simulink model "waterTankBurner"  (R2014b)
settings: Solver=ode1  StartTime=0.0  StopTime=100  FixedStep=0.0001  MaxStep=0.0001  RelTol=1e-3
(part 1 of 4)
settings Model: Creator=sand080  LastModifiedBy=nall426
settings DataIOCC: LimitDataPoints=off
settings RTWCC: CustomInitializer=gettimeofday(&t0, 0);
settings RTWCC: CustomSourceCode=|
  | int gettimeofday(struct timeval * tp, struct timezone * tzp)
  | {
  |     // Note: some broken versions only have 8 trailing zero's, the correct epoch has 9 trailing zero's
  |     static const uint64_t EPOCH = ((uint64_t) 116444736000000000ULL);
  | 
  |     SYSTEMTIME  system_time;
  |     FILETIME    file_time;
  |     uint64_t    time;
  | 
  | 	GetSystemTime( &system_time );
  |     SystemTimeToFileTime( &system_time, &file_time );
  |     time =  ((uint64_t)file_time.dwLowDateTime )      ;
  |     time += ((uint64_t)file_time.dwHighDateTime) << 32;
  | 
  |     tp->tv_sec  = (long) ((time - EPOCH) / 10000000L);
  |     tp->tv_usec = (long) (system_time.wMilliseconds * 1000);
  |     return 0;
  | }
  | 
  | struct timeval t0, t1;
settings RTWCC: CustomHeaderCode=|
  | #include <stdint.h> // portable: uint64_t   MSVC: __int64
  | #include <Windows.h>
settings RTWCC: CustomTerminator=|
  | gettimeofday(&t1, 0);
  | 
  | long elapsed = (t1.tv_sec-t0.tv_sec)*1000000 + t1.tv_usec-t0.tv_usec;
  | printf("Time taken: %ld microseconds (%.3f seconds)\n", elapsed, (elapsed / 1000000.0));

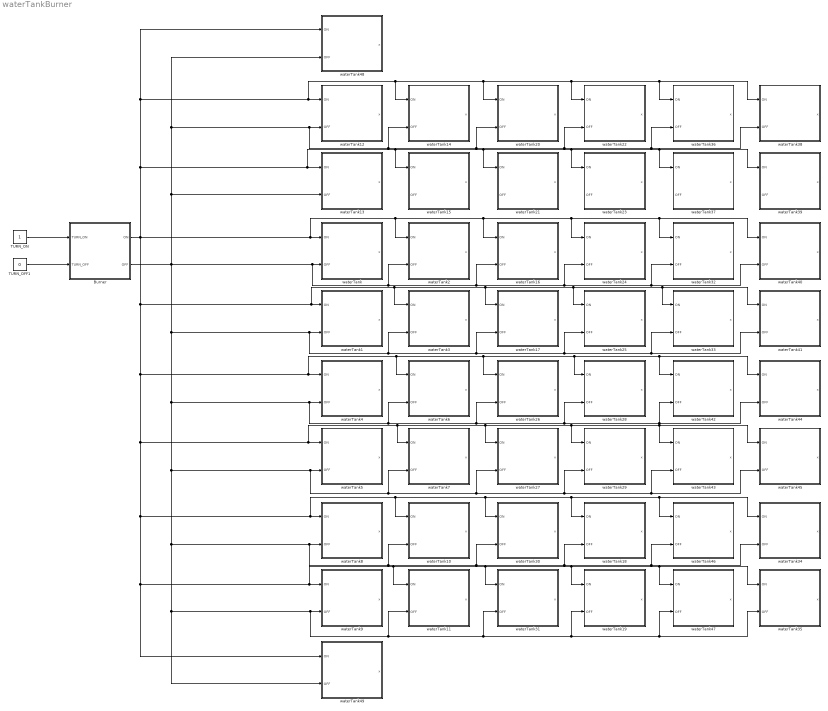
== system waterTankBurner ==
  Burner : Subsystem
  TURN_OFF1 : Constant  Value=0
  TURN_ON : Constant
  waterTank : Subsystem
  waterTank1 : Subsystem
  waterTank10 : Subsystem
  waterTank11 : Subsystem
  waterTank12 : Subsystem
  waterTank13 : Subsystem
  waterTank14 : Subsystem
  waterTank15 : Subsystem
  waterTank16 : Subsystem
  waterTank17 : Subsystem
  waterTank18 : Subsystem
  waterTank19 : Subsystem
  waterTank2 : Subsystem
  waterTank20 : Subsystem
  waterTank21 : Subsystem
  waterTank22 : Subsystem
  waterTank23 : Subsystem
  waterTank24 : Subsystem
  waterTank25 : Subsystem
  waterTank26 : Subsystem
  waterTank27 : Subsystem
  waterTank28 : Subsystem
  waterTank29 : Subsystem
  waterTank3 : Subsystem
  waterTank30 : Subsystem
  waterTank31 : Subsystem
  waterTank32 : Subsystem
  waterTank33 : Subsystem
  waterTank34 : Subsystem
  waterTank35 : Subsystem
  waterTank36 : Subsystem
  waterTank37 : Subsystem
  waterTank38 : Subsystem
  waterTank39 : Subsystem
  waterTank4 : Subsystem
  waterTank40 : Subsystem
  waterTank41 : Subsystem
  waterTank42 : Subsystem
  waterTank43 : Subsystem
  waterTank44 : Subsystem
  waterTank45 : Subsystem
  waterTank46 : Subsystem
  waterTank47 : Subsystem
  waterTank48 : Subsystem
  waterTank49 : Subsystem
  waterTank5 : Subsystem
  waterTank6 : Subsystem
  waterTank7 : Subsystem
  waterTank8 : Subsystem
  waterTank9 : Subsystem
  wires:
  TURN_ON/1 -> Burner/1(TURN_ON)
  TURN_OFF1/1 -> Burner/2(TURN_OFF)
  Burner/1(ON) -> waterTank38/1(ON), waterTank36/1(ON), waterTank22/1(ON), waterTank20/1(ON), waterTank14/1(ON), waterTank12/1(ON), waterTank48/1(ON), waterTank39/1(ON), waterTank37/1(ON), waterTank23/1(ON), waterTank21/1(ON), waterTank15/1(ON), waterTank13/1(ON), waterTank49/1(ON), waterTank11/1(ON), waterTank31/1(ON), waterTank19/1(ON), waterTank47/1(ON), waterTank35/1(ON), waterTank9/1(ON), waterTank10/1(ON), waterTank30/1(ON), waterTank18/1(ON), waterTank46/1(ON), waterTank34/1(ON), waterTank8/1(ON), waterTank7/1(ON), waterTank27/1(ON), waterTank29/1(ON), waterTank43/1(ON), waterTank45/1(ON), waterTank5/1(ON), waterTank6/1(ON), waterTank26/1(ON), waterTank28/1(ON), waterTank42/1(ON), waterTank44/1(ON), waterTank4/1(ON), waterTank3/1(ON), waterTank25/1(ON), waterTank33/1(ON), waterTank41/1(ON), waterTank17/1(ON), waterTank1/1(ON), waterTank40/1(ON), waterTank32/1(ON), waterTank24/1(ON), waterTank16/1(ON), waterTank2/1(ON), waterTank/1(ON)
  Burner/2(OFF) -> waterTank48/2(OFF), waterTank36/2(OFF), waterTank38/2(OFF), waterTank22/2(OFF), waterTank20/2(OFF), waterTank14/2(OFF), waterTank12/2(OFF), waterTank13/2(OFF), waterTank49/2(OFF), waterTank19/2(OFF), waterTank47/2(OFF), waterTank35/2(OFF), waterTank31/2(OFF), waterTank11/2(OFF), waterTank9/2(OFF), waterTank46/2(OFF), waterTank34/2(OFF), waterTank18/2(OFF), waterTank30/2(OFF), waterTank10/2(OFF), waterTank8/2(OFF), waterTank43/2(OFF), waterTank45/2(OFF), waterTank29/2(OFF), waterTank27/2(OFF), waterTank7/2(OFF), waterTank5/2(OFF), waterTank42/2(OFF), waterTank44/2(OFF), waterTank28/2(OFF), waterTank26/2(OFF), waterTank6/2(OFF), waterTank4/2(OFF), waterTank33/2(OFF), waterTank41/2(OFF), waterTank25/2(OFF), waterTank17/2(OFF), waterTank3/2(OFF), waterTank1/2(OFF), waterTank16/2(OFF), waterTank40/2(OFF), waterTank32/2(OFF), waterTank24/2(OFF), waterTank2/2(OFF), waterTank/2(OFF)

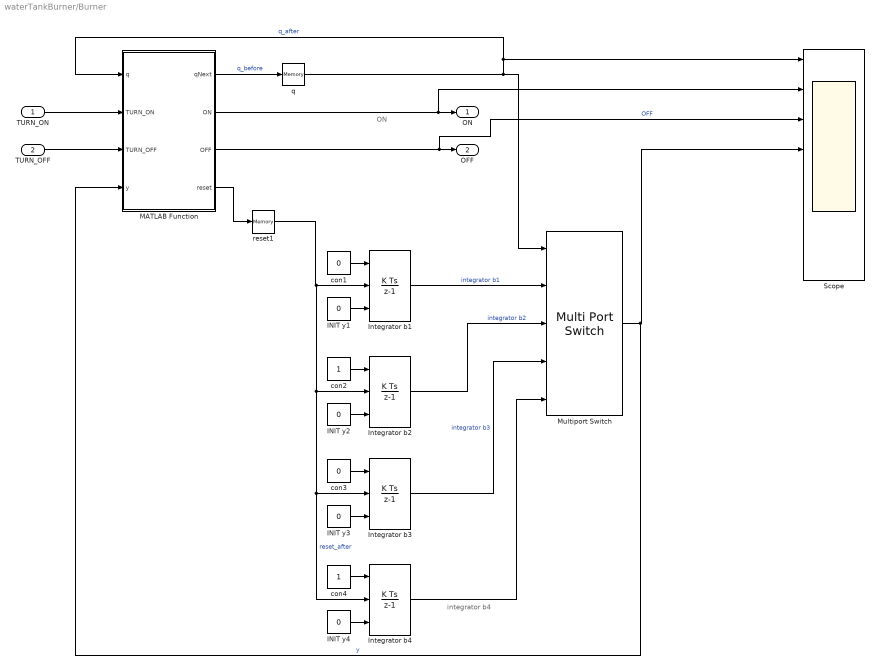
== system waterTankBurner/Burner ==
  note: integrator b4
  note: ON
  TURN_ON : Inport
  TURN_OFF : Inport  Port=2
  INIT y{1..4} (4 alike) : Constant  Value=0
  Integrator b{1..4} (4 alike) : DiscreteIntegrator  ExternalReset=either  InitialConditionSource=external  InitialCondition=510  InitialConditionSetting=State (most efficient)  SampleTime=-1
  MATLAB Function : MATLAB Function  Priority=1  TreatAsAtomicUnit=on
  Multiport Switch : MultiPortSwitch  Inputs=4
  Scope : Scope  NumInputPorts=8
      settings: TickLabels=on  ShowLegends=on  YMin=0~0~0~0~0~0~0~0  YMax=1~1~1~1~1~1~1~1
  con1 : Constant  Value=0
  con2 : Constant
  con3 : Constant  Value=0
  con4 : Constant
  q : Memory  X0=1  LinearizeMemory=on
  reset1 : Memory  LinearizeMemory=on
  ON : Outport
  OFF : Outport  Port=2
  wires:
  MATLAB Function/3(OFF) -> Scope/3, OFF/1  "OFF"
  INIT y1/1 -> Integrator b1/3
  INIT y2/1 -> Integrator b2/3
  con1/1 -> Integrator b1/1
  MATLAB Function/1(qNext) -> q/1  "q_before"
  q/1 -> Multiport Switch/1, MATLAB Function/1(q), Scope/1  "q_after"
  MATLAB Function/4(reset) -> reset1/1
  con2/1 -> Integrator b2/1
  MATLAB Function/2(ON) -> Scope/2, ON/1
  TURN_OFF/1 -> MATLAB Function/3(TURN_OFF)
  TURN_ON/1 -> MATLAB Function/2(TURN_ON)
  INIT y3/1 -> Integrator b3/3
  INIT y4/1 -> Integrator b4/3
  con3/1 -> Integrator b3/1
  con4/1 -> Integrator b4/1
  reset1/1 -> Integrator b4/2, Integrator b3/2, Integrator b2/2, Integrator b1/2  "reset_after"
  Integrator b1/1 -> Multiport Switch/2  "integrator b1"
  Integrator b2/1 -> Multiport Switch/3  "integrator b2"
  Integrator b3/1 -> Multiport Switch/4  "integrator b3"
  Integrator b4/1 -> Multiport Switch/5
  Multiport Switch/1 -> MATLAB Function/4(y), Scope/4  "y"

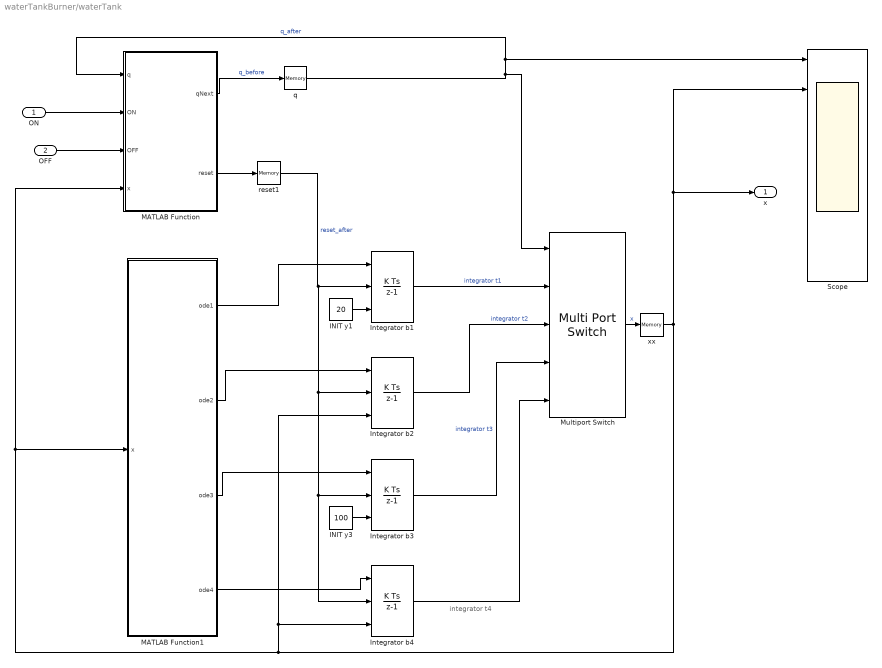
== system waterTankBurner/waterTank ==
  note: integrator t4
  ON : Inport
  OFF : Inport  Port=2
  INIT y1 : Constant  Value=20
  INIT y3 : Constant  Value=100
  Integrator b{1..4} (4 alike) : DiscreteIntegrator  ExternalReset=either  InitialConditionSource=external  InitialCondition=510  InitialConditionSetting=State (most efficient)  SampleTime=-1
  MATLAB Function : MATLAB Function  Priority=1  TreatAsAtomicUnit=on
  MATLAB Function1 : MATLAB Function  TreatAsAtomicUnit=on
  Multiport Switch : MultiPortSwitch  Inputs=4
  Scope : Scope  NumInputPorts=8
      settings: TickLabels=on  ShowLegends=on  YMin=0~0~0~0~0~0~0~0  YMax=1~1~1~1~1~1~1~1
  q : Memory  X0=1  LinearizeMemory=on
  reset1 : Memory  LinearizeMemory=on
  xx : Memory  LinearizeMemory=on
  x : Outport
  wires:
  INIT y1/1 -> Integrator b1/3
  MATLAB Function1/1(ode1) -> Integrator b1/1
  MATLAB Function/1(qNext) -> q/1  "q_before"
  q/1 -> Multiport Switch/1, MATLAB Function/1(q), Scope/1  "q_after"
  MATLAB Function/2(reset) -> reset1/1
  MATLAB Function1/2(ode2) -> Integrator b2/1
  INIT y3/1 -> Integrator b3/3
  MATLAB Function1/3(ode3) -> Integrator b3/1
  MATLAB Function1/4(ode4) -> Integrator b4/1
  reset1/1 -> Integrator b4/2, Integrator b3/2, Integrator b2/2, Integrator b1/2  "reset_after"
  Integrator b1/1 -> Multiport Switch/2  "integrator t1"
  Integrator b2/1 -> Multiport Switch/3  "integrator t2"
  Integrator b3/1 -> Multiport Switch/4  "integrator t3"
  Integrator b4/1 -> Multiport Switch/5
  OFF/1 -> MATLAB Function/3(OFF)
  ON/1 -> MATLAB Function/2(ON)
  xx/1 -> x/1, Scope/2, Integrator b2/3, Integrator b4/3, MATLAB Function1/1(x), MATLAB Function/4(x)
  Multiport Switch/1 -> xx/1  "x"

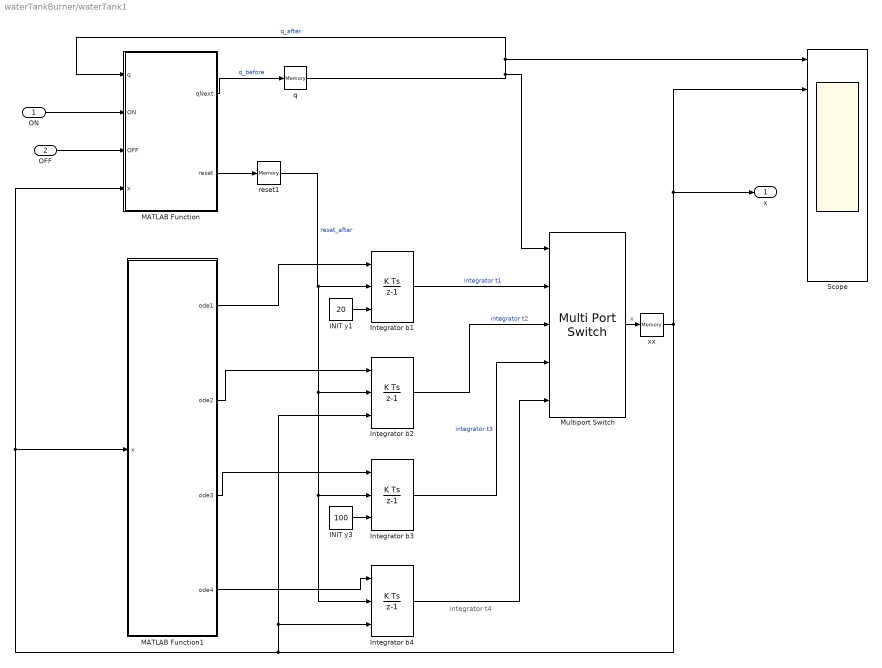
== system waterTankBurner/waterTank1 ==
  note: integrator t4
  ON : Inport
  OFF : Inport  Port=2
  INIT y1 : Constant  Value=20
  INIT y3 : Constant  Value=100
  Integrator b{1..4} (4 alike) : DiscreteIntegrator  ExternalReset=either  InitialConditionSource=external  InitialCondition=510  InitialConditionSetting=State (most efficient)  SampleTime=-1
  MATLAB Function : MATLAB Function  Priority=1  TreatAsAtomicUnit=on
  MATLAB Function1 : MATLAB Function  TreatAsAtomicUnit=on
  Multiport Switch : MultiPortSwitch  Inputs=4
  Scope : Scope  NumInputPorts=8
      settings: TickLabels=on  ShowLegends=on  YMin=0~0~0~0~0~0~0~0  YMax=1~1~1~1~1~1~1~1
  q : Memory  X0=1  LinearizeMemory=on
  reset1 : Memory  LinearizeMemory=on
  xx : Memory  LinearizeMemory=on
  x : Outport
  wires:
  INIT y1/1 -> Integrator b1/3
  MATLAB Function1/1(ode1) -> Integrator b1/1
  MATLAB Function/1(qNext) -> q/1  "q_before"
  q/1 -> Multiport Switch/1, MATLAB Function/1(q), Scope/1  "q_after"
  MATLAB Function/2(reset) -> reset1/1
  MATLAB Function1/2(ode2) -> Integrator b2/1
  INIT y3/1 -> Integrator b3/3
  MATLAB Function1/3(ode3) -> Integrator b3/1
  MATLAB Function1/4(ode4) -> Integrator b4/1
  reset1/1 -> Integrator b4/2, Integrator b3/2, Integrator b2/2, Integrator b1/2  "reset_after"
  Integrator b1/1 -> Multiport Switch/2  "integrator t1"
  Integrator b2/1 -> Multiport Switch/3  "integrator t2"
  Integrator b3/1 -> Multiport Switch/4  "integrator t3"
  Integrator b4/1 -> Multiport Switch/5
  OFF/1 -> MATLAB Function/3(OFF)
  ON/1 -> MATLAB Function/2(ON)
  xx/1 -> x/1, Scope/2, Integrator b2/3, Integrator b4/3, MATLAB Function1/1(x), MATLAB Function/4(x)
  Multiport Switch/1 -> xx/1  "x"

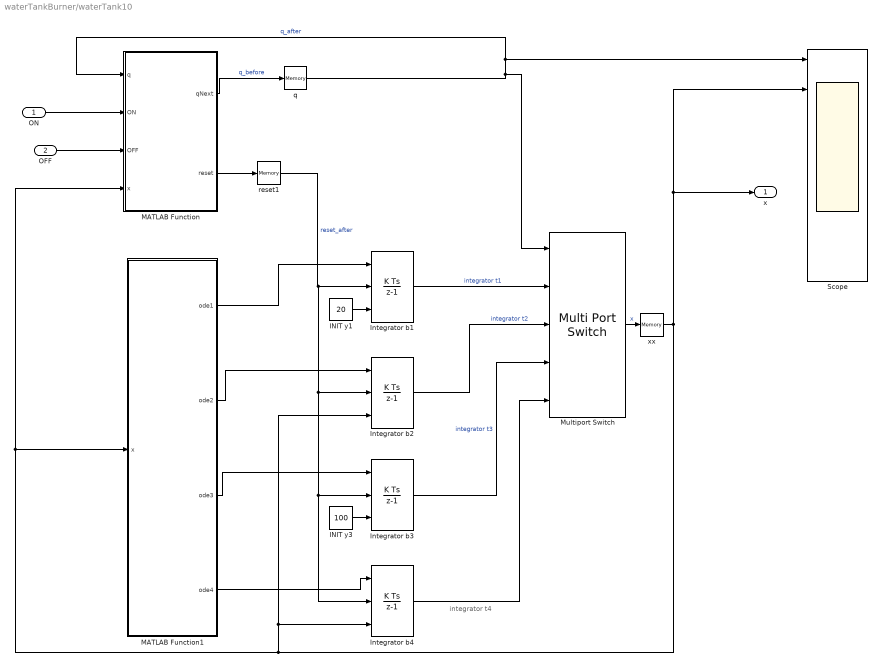
== system waterTankBurner/waterTank10 ==
  note: integrator t4
  ON : Inport
  OFF : Inport  Port=2
  INIT y1 : Constant  Value=20
  INIT y3 : Constant  Value=100
  Integrator b{1..4} (4 alike) : DiscreteIntegrator  ExternalReset=either  InitialConditionSource=external  InitialCondition=510  InitialConditionSetting=State (most efficient)  SampleTime=-1
  MATLAB Function : MATLAB Function  Priority=1  TreatAsAtomicUnit=on
  MATLAB Function1 : MATLAB Function  TreatAsAtomicUnit=on
  Multiport Switch : MultiPortSwitch  Inputs=4
  Scope : Scope  NumInputPorts=8
      settings: TickLabels=on  ShowLegends=on  YMin=0~0~0~0~0~0~0~0  YMax=1~1~1~1~1~1~1~1
  q : Memory  X0=1  LinearizeMemory=on
  reset1 : Memory  LinearizeMemory=on
  xx : Memory  LinearizeMemory=on
  x : Outport
  wires:
  INIT y1/1 -> Integrator b1/3
  MATLAB Function1/1(ode1) -> Integrator b1/1
  MATLAB Function/1(qNext) -> q/1  "q_before"
  q/1 -> Multiport Switch/1, MATLAB Function/1(q), Scope/1  "q_after"
  MATLAB Function/2(reset) -> reset1/1
  MATLAB Function1/2(ode2) -> Integrator b2/1
  INIT y3/1 -> Integrator b3/3
  MATLAB Function1/3(ode3) -> Integrator b3/1
  MATLAB Function1/4(ode4) -> Integrator b4/1
  reset1/1 -> Integrator b4/2, Integrator b3/2, Integrator b2/2, Integrator b1/2  "reset_after"
  Integrator b1/1 -> Multiport Switch/2  "integrator t1"
  Integrator b2/1 -> Multiport Switch/3  "integrator t2"
  Integrator b3/1 -> Multiport Switch/4  "integrator t3"
  Integrator b4/1 -> Multiport Switch/5
  OFF/1 -> MATLAB Function/3(OFF)
  ON/1 -> MATLAB Function/2(ON)
  xx/1 -> x/1, Scope/2, Integrator b2/3, Integrator b4/3, MATLAB Function1/1(x), MATLAB Function/4(x)
  Multiport Switch/1 -> xx/1  "x"

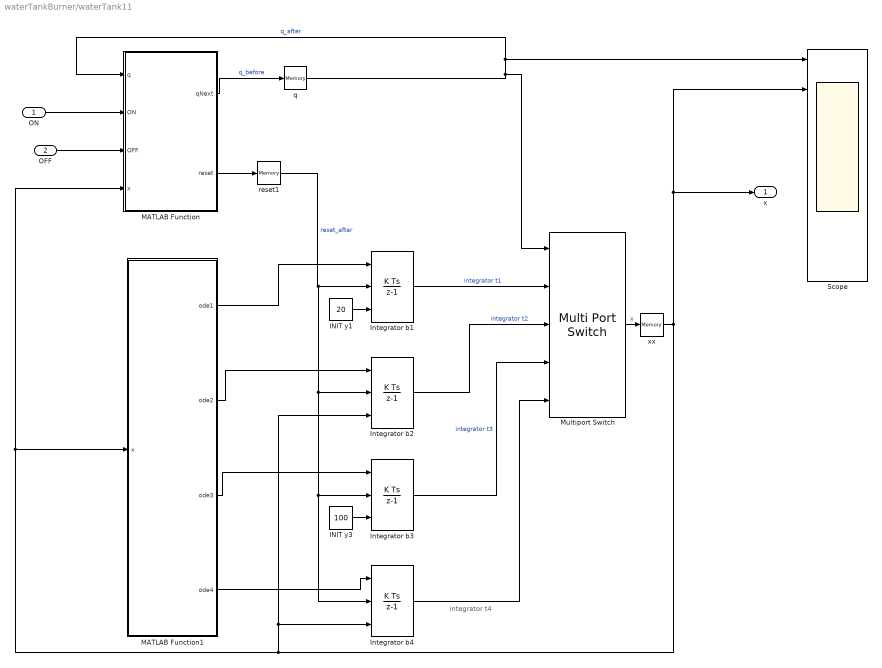
== system waterTankBurner/waterTank11 ==
  note: integrator t4
  ON : Inport
  OFF : Inport  Port=2
  INIT y1 : Constant  Value=20
  INIT y3 : Constant  Value=100
  Integrator b{1..4} (4 alike) : DiscreteIntegrator  ExternalReset=either  InitialConditionSource=external  InitialCondition=510  InitialConditionSetting=State (most efficient)  SampleTime=-1
  MATLAB Function : MATLAB Function  Priority=1  TreatAsAtomicUnit=on
  MATLAB Function1 : MATLAB Function  TreatAsAtomicUnit=on
  Multiport Switch : MultiPortSwitch  Inputs=4
  Scope : Scope  NumInputPorts=8
      settings: TickLabels=on  ShowLegends=on  YMin=0~0~0~0~0~0~0~0  YMax=1~1~1~1~1~1~1~1
  q : Memory  X0=1  LinearizeMemory=on
  reset1 : Memory  LinearizeMemory=on
  xx : Memory  LinearizeMemory=on
  x : Outport
  wires:
  INIT y1/1 -> Integrator b1/3
  MATLAB Function1/1(ode1) -> Integrator b1/1
  MATLAB Function/1(qNext) -> q/1  "q_before"
  q/1 -> Multiport Switch/1, MATLAB Function/1(q), Scope/1  "q_after"
  MATLAB Function/2(reset) -> reset1/1
  MATLAB Function1/2(ode2) -> Integrator b2/1
  INIT y3/1 -> Integrator b3/3
  MATLAB Function1/3(ode3) -> Integrator b3/1
  MATLAB Function1/4(ode4) -> Integrator b4/1
  reset1/1 -> Integrator b4/2, Integrator b3/2, Integrator b2/2, Integrator b1/2  "reset_after"
  Integrator b1/1 -> Multiport Switch/2  "integrator t1"
  Integrator b2/1 -> Multiport Switch/3  "integrator t2"
  Integrator b3/1 -> Multiport Switch/4  "integrator t3"
  Integrator b4/1 -> Multiport Switch/5
  OFF/1 -> MATLAB Function/3(OFF)
  ON/1 -> MATLAB Function/2(ON)
  xx/1 -> x/1, Scope/2, Integrator b2/3, Integrator b4/3, MATLAB Function1/1(x), MATLAB Function/4(x)
  Multiport Switch/1 -> xx/1  "x"

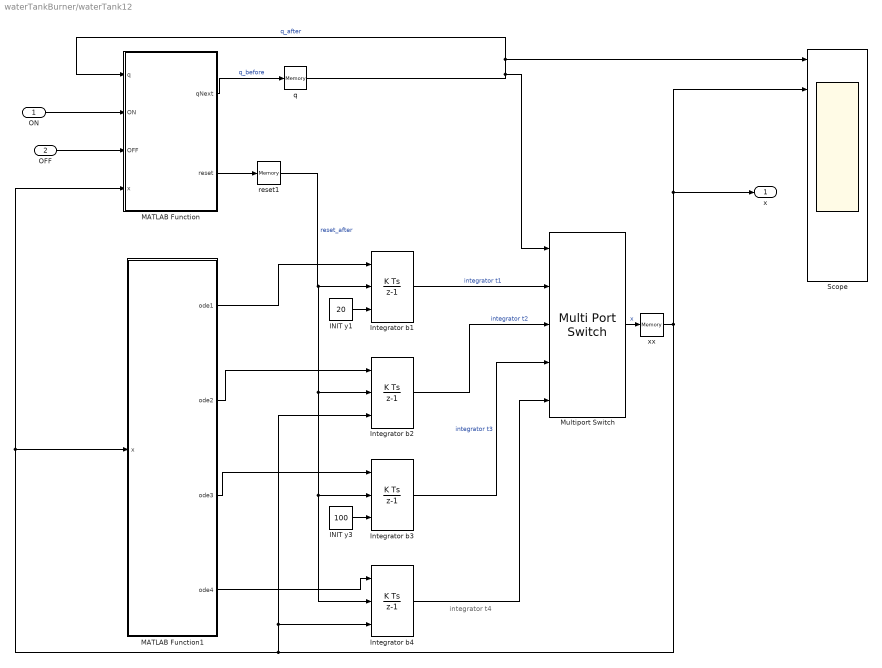
== system waterTankBurner/waterTank12 ==
  note: integrator t4
  ON : Inport
  OFF : Inport  Port=2
  INIT y1 : Constant  Value=20
  INIT y3 : Constant  Value=100
  Integrator b{1..4} (4 alike) : DiscreteIntegrator  ExternalReset=either  InitialConditionSource=external  InitialCondition=510  InitialConditionSetting=State (most efficient)  SampleTime=-1
  MATLAB Function : MATLAB Function  Priority=1  TreatAsAtomicUnit=on
  MATLAB Function1 : MATLAB Function  TreatAsAtomicUnit=on
  Multiport Switch : MultiPortSwitch  Inputs=4
  Scope : Scope  NumInputPorts=8
      settings: TickLabels=on  ShowLegends=on  YMin=0~0~0~0~0~0~0~0  YMax=1~1~1~1~1~1~1~1
  q : Memory  X0=1  LinearizeMemory=on
  reset1 : Memory  LinearizeMemory=on
  xx : Memory  LinearizeMemory=on
  x : Outport
  wires:
  INIT y1/1 -> Integrator b1/3
  MATLAB Function1/1(ode1) -> Integrator b1/1
  MATLAB Function/1(qNext) -> q/1  "q_before"
  q/1 -> Multiport Switch/1, MATLAB Function/1(q), Scope/1  "q_after"
  MATLAB Function/2(reset) -> reset1/1
  MATLAB Function1/2(ode2) -> Integrator b2/1
  INIT y3/1 -> Integrator b3/3
  MATLAB Function1/3(ode3) -> Integrator b3/1
  MATLAB Function1/4(ode4) -> Integrator b4/1
  reset1/1 -> Integrator b4/2, Integrator b3/2, Integrator b2/2, Integrator b1/2  "reset_after"
  Integrator b1/1 -> Multiport Switch/2  "integrator t1"
  Integrator b2/1 -> Multiport Switch/3  "integrator t2"
  Integrator b3/1 -> Multiport Switch/4  "integrator t3"
  Integrator b4/1 -> Multiport Switch/5
  OFF/1 -> MATLAB Function/3(OFF)
  ON/1 -> MATLAB Function/2(ON)
  xx/1 -> x/1, Scope/2, Integrator b2/3, Integrator b4/3, MATLAB Function1/1(x), MATLAB Function/4(x)
  Multiport Switch/1 -> xx/1  "x"

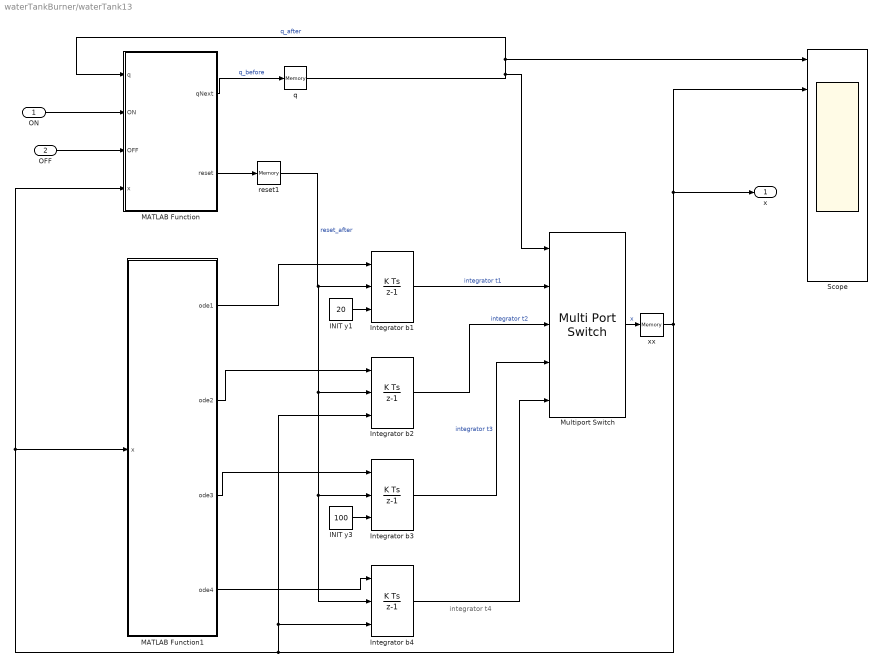
== system waterTankBurner/waterTank13 ==
  note: integrator t4
  ON : Inport
  OFF : Inport  Port=2
  INIT y1 : Constant  Value=20
  INIT y3 : Constant  Value=100
  Integrator b{1..4} (4 alike) : DiscreteIntegrator  ExternalReset=either  InitialConditionSource=external  InitialCondition=510  InitialConditionSetting=State (most efficient)  SampleTime=-1
  MATLAB Function : MATLAB Function  Priority=1  TreatAsAtomicUnit=on
  MATLAB Function1 : MATLAB Function  TreatAsAtomicUnit=on
  Multiport Switch : MultiPortSwitch  Inputs=4
  Scope : Scope  NumInputPorts=8
      settings: TickLabels=on  ShowLegends=on  YMin=0~0~0~0~0~0~0~0  YMax=1~1~1~1~1~1~1~1
  q : Memory  X0=1  LinearizeMemory=on
  reset1 : Memory  LinearizeMemory=on
  xx : Memory  LinearizeMemory=on
  x : Outport
  wires:
  INIT y1/1 -> Integrator b1/3
  MATLAB Function1/1(ode1) -> Integrator b1/1
  MATLAB Function/1(qNext) -> q/1  "q_before"
  q/1 -> Multiport Switch/1, MATLAB Function/1(q), Scope/1  "q_after"
  MATLAB Function/2(reset) -> reset1/1
  MATLAB Function1/2(ode2) -> Integrator b2/1
  INIT y3/1 -> Integrator b3/3
  MATLAB Function1/3(ode3) -> Integrator b3/1
  MATLAB Function1/4(ode4) -> Integrator b4/1
  reset1/1 -> Integrator b4/2, Integrator b3/2, Integrator b2/2, Integrator b1/2  "reset_after"
  Integrator b1/1 -> Multiport Switch/2  "integrator t1"
  Integrator b2/1 -> Multiport Switch/3  "integrator t2"
  Integrator b3/1 -> Multiport Switch/4  "integrator t3"
  Integrator b4/1 -> Multiport Switch/5
  OFF/1 -> MATLAB Function/3(OFF)
  ON/1 -> MATLAB Function/2(ON)
  xx/1 -> x/1, Scope/2, Integrator b2/3, Integrator b4/3, MATLAB Function1/1(x), MATLAB Function/4(x)
  Multiport Switch/1 -> xx/1  "x"

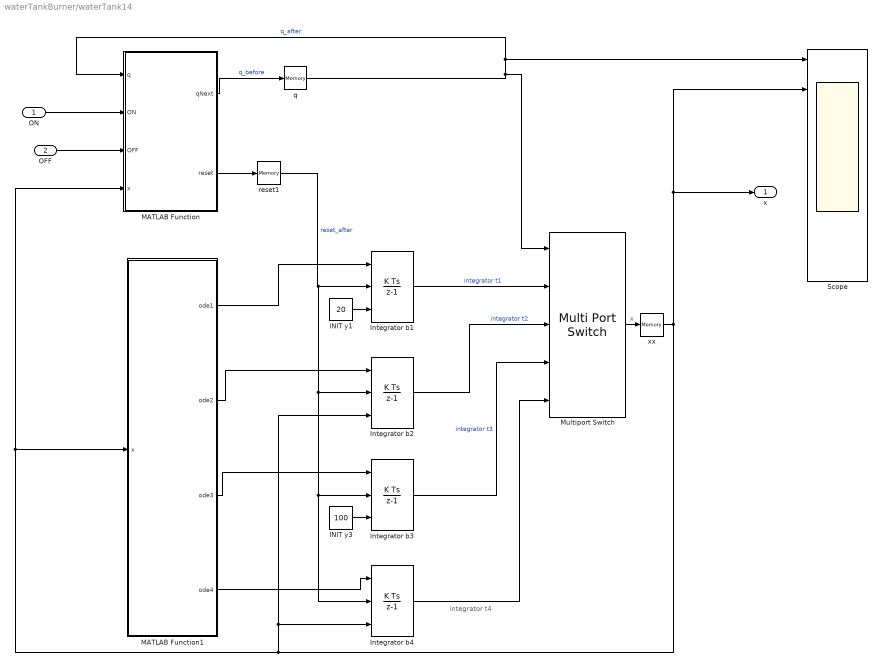
== system waterTankBurner/waterTank14 ==
  note: integrator t4
  ON : Inport
  OFF : Inport  Port=2
  INIT y1 : Constant  Value=20
  INIT y3 : Constant  Value=100
  Integrator b{1..4} (4 alike) : DiscreteIntegrator  ExternalReset=either  InitialConditionSource=external  InitialCondition=510  InitialConditionSetting=State (most efficient)  SampleTime=-1
  MATLAB Function : MATLAB Function  Priority=1  TreatAsAtomicUnit=on
  MATLAB Function1 : MATLAB Function  TreatAsAtomicUnit=on
  Multiport Switch : MultiPortSwitch  Inputs=4
  Scope : Scope  NumInputPorts=8
      settings: TickLabels=on  ShowLegends=on  YMin=0~0~0~0~0~0~0~0  YMax=1~1~1~1~1~1~1~1
  q : Memory  X0=1  LinearizeMemory=on
  reset1 : Memory  LinearizeMemory=on
  xx : Memory  LinearizeMemory=on
  x : Outport
  wires:
  INIT y1/1 -> Integrator b1/3
  MATLAB Function1/1(ode1) -> Integrator b1/1
  MATLAB Function/1(qNext) -> q/1  "q_before"
  q/1 -> Multiport Switch/1, MATLAB Function/1(q), Scope/1  "q_after"
  MATLAB Function/2(reset) -> reset1/1
  MATLAB Function1/2(ode2) -> Integrator b2/1
  INIT y3/1 -> Integrator b3/3
  MATLAB Function1/3(ode3) -> Integrator b3/1
  MATLAB Function1/4(ode4) -> Integrator b4/1
  reset1/1 -> Integrator b4/2, Integrator b3/2, Integrator b2/2, Integrator b1/2  "reset_after"
  Integrator b1/1 -> Multiport Switch/2  "integrator t1"
  Integrator b2/1 -> Multiport Switch/3  "integrator t2"
  Integrator b3/1 -> Multiport Switch/4  "integrator t3"
  Integrator b4/1 -> Multiport Switch/5
  OFF/1 -> MATLAB Function/3(OFF)
  ON/1 -> MATLAB Function/2(ON)
  xx/1 -> x/1, Scope/2, Integrator b2/3, Integrator b4/3, MATLAB Function1/1(x), MATLAB Function/4(x)
  Multiport Switch/1 -> xx/1  "x"

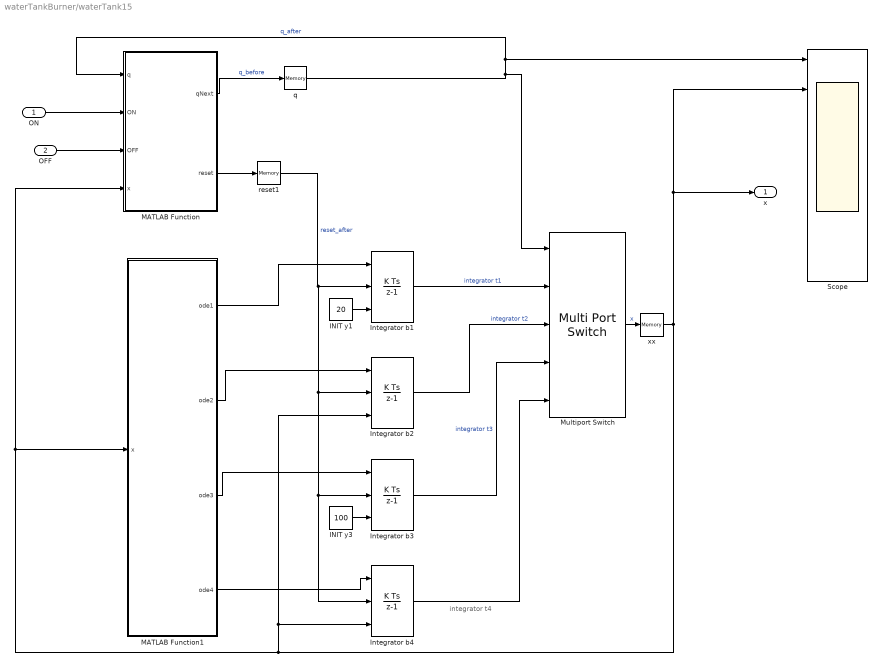
== system waterTankBurner/waterTank15 ==
  note: integrator t4
  ON : Inport
  OFF : Inport  Port=2
  INIT y1 : Constant  Value=20
  INIT y3 : Constant  Value=100
  Integrator b{1..4} (4 alike) : DiscreteIntegrator  ExternalReset=either  InitialConditionSource=external  InitialCondition=510  InitialConditionSetting=State (most efficient)  SampleTime=-1
  MATLAB Function : MATLAB Function  Priority=1  TreatAsAtomicUnit=on
  MATLAB Function1 : MATLAB Function  TreatAsAtomicUnit=on
  Multiport Switch : MultiPortSwitch  Inputs=4
  Scope : Scope  NumInputPorts=8
      settings: TickLabels=on  ShowLegends=on  YMin=0~0~0~0~0~0~0~0  YMax=1~1~1~1~1~1~1~1
  q : Memory  X0=1  LinearizeMemory=on
  reset1 : Memory  LinearizeMemory=on
  xx : Memory  LinearizeMemory=on
  x : Outport
  wires:
  INIT y1/1 -> Integrator b1/3
  MATLAB Function1/1(ode1) -> Integrator b1/1
  MATLAB Function/1(qNext) -> q/1  "q_before"
  q/1 -> Multiport Switch/1, MATLAB Function/1(q), Scope/1  "q_after"
  MATLAB Function/2(reset) -> reset1/1
  MATLAB Function1/2(ode2) -> Integrator b2/1
  INIT y3/1 -> Integrator b3/3
  MATLAB Function1/3(ode3) -> Integrator b3/1
  MATLAB Function1/4(ode4) -> Integrator b4/1
  reset1/1 -> Integrator b4/2, Integrator b3/2, Integrator b2/2, Integrator b1/2  "reset_after"
  Integrator b1/1 -> Multiport Switch/2  "integrator t1"
  Integrator b2/1 -> Multiport Switch/3  "integrator t2"
  Integrator b3/1 -> Multiport Switch/4  "integrator t3"
  Integrator b4/1 -> Multiport Switch/5
  OFF/1 -> MATLAB Function/3(OFF)
  ON/1 -> MATLAB Function/2(ON)
  xx/1 -> x/1, Scope/2, Integrator b2/3, Integrator b4/3, MATLAB Function1/1(x), MATLAB Function/4(x)
  Multiport Switch/1 -> xx/1  "x"

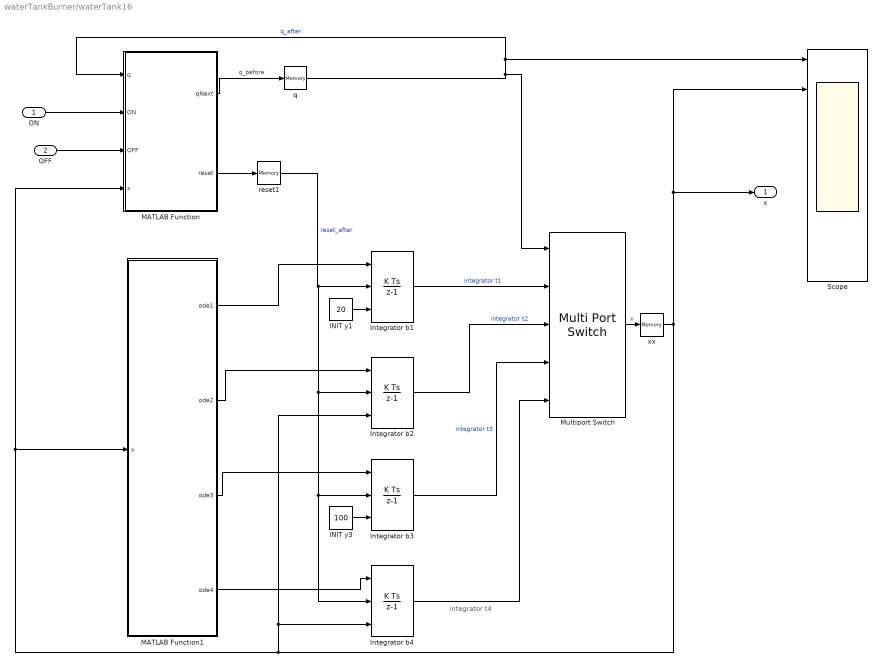
== system waterTankBurner/waterTank16 ==
  note: integrator t4
  ON : Inport
  OFF : Inport  Port=2
  INIT y1 : Constant  Value=20
  INIT y3 : Constant  Value=100
  Integrator b{1..4} (4 alike) : DiscreteIntegrator  ExternalReset=either  InitialConditionSource=external  InitialCondition=510  InitialConditionSetting=State (most efficient)  SampleTime=-1
  MATLAB Function : MATLAB Function  Priority=1  TreatAsAtomicUnit=on
  MATLAB Function1 : MATLAB Function  TreatAsAtomicUnit=on
  Multiport Switch : MultiPortSwitch  Inputs=4
  Scope : Scope  NumInputPorts=8
      settings: TickLabels=on  ShowLegends=on  YMin=0~0~0~0~0~0~0~0  YMax=1~1~1~1~1~1~1~1
  q : Memory  X0=1  LinearizeMemory=on
  reset1 : Memory  LinearizeMemory=on
  xx : Memory  LinearizeMemory=on
  x : Outport
  wires:
  INIT y1/1 -> Integrator b1/3
  MATLAB Function1/1(ode1) -> Integrator b1/1
  MATLAB Function/1(qNext) -> q/1  "q_before"
  q/1 -> Multiport Switch/1, MATLAB Function/1(q), Scope/1  "q_after"
  MATLAB Function/2(reset) -> reset1/1
  MATLAB Function1/2(ode2) -> Integrator b2/1
  INIT y3/1 -> Integrator b3/3
  MATLAB Function1/3(ode3) -> Integrator b3/1
  MATLAB Function1/4(ode4) -> Integrator b4/1
  reset1/1 -> Integrator b4/2, Integrator b3/2, Integrator b2/2, Integrator b1/2  "reset_after"
  Integrator b1/1 -> Multiport Switch/2  "integrator t1"
  Integrator b2/1 -> Multiport Switch/3  "integrator t2"
  Integrator b3/1 -> Multiport Switch/4  "integrator t3"
  Integrator b4/1 -> Multiport Switch/5
  OFF/1 -> MATLAB Function/3(OFF)
  ON/1 -> MATLAB Function/2(ON)
  xx/1 -> x/1, Scope/2, Integrator b2/3, Integrator b4/3, MATLAB Function1/1(x), MATLAB Function/4(x)
  Multiport Switch/1 -> xx/1  "x"

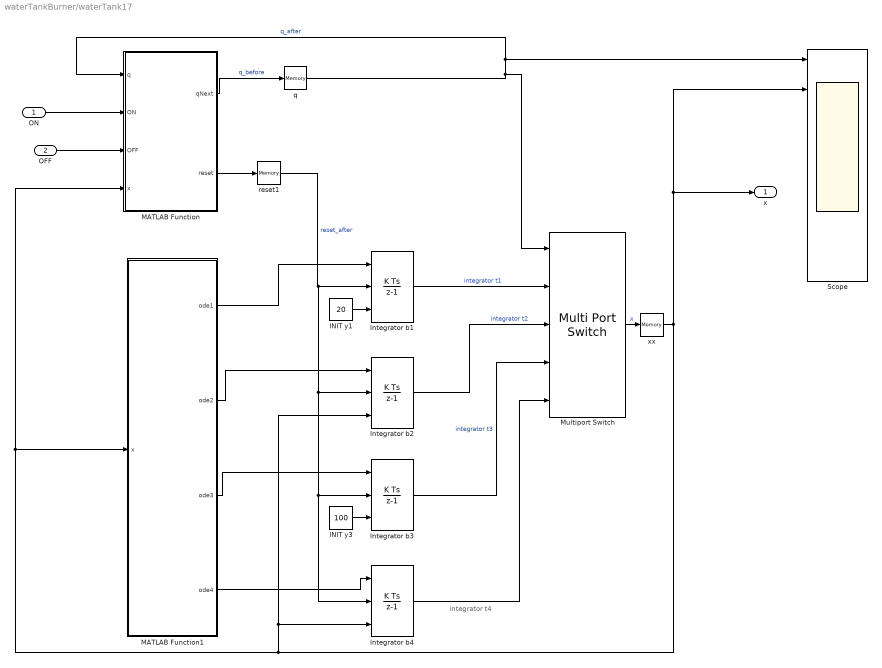
== system waterTankBurner/waterTank17 ==
  note: integrator t4
  ON : Inport
  OFF : Inport  Port=2
  INIT y1 : Constant  Value=20
  INIT y3 : Constant  Value=100
  Integrator b{1..4} (4 alike) : DiscreteIntegrator  ExternalReset=either  InitialConditionSource=external  InitialCondition=510  InitialConditionSetting=State (most efficient)  SampleTime=-1
  MATLAB Function : MATLAB Function  Priority=1  TreatAsAtomicUnit=on
  MATLAB Function1 : MATLAB Function  TreatAsAtomicUnit=on
  Multiport Switch : MultiPortSwitch  Inputs=4
  Scope : Scope  NumInputPorts=8
      settings: TickLabels=on  ShowLegends=on  YMin=0~0~0~0~0~0~0~0  YMax=1~1~1~1~1~1~1~1
  q : Memory  X0=1  LinearizeMemory=on
  reset1 : Memory  LinearizeMemory=on
  xx : Memory  LinearizeMemory=on
  x : Outport
  wires:
  INIT y1/1 -> Integrator b1/3
  MATLAB Function1/1(ode1) -> Integrator b1/1
  MATLAB Function/1(qNext) -> q/1  "q_before"
  q/1 -> Multiport Switch/1, MATLAB Function/1(q), Scope/1  "q_after"
  MATLAB Function/2(reset) -> reset1/1
  MATLAB Function1/2(ode2) -> Integrator b2/1
  INIT y3/1 -> Integrator b3/3
  MATLAB Function1/3(ode3) -> Integrator b3/1
  MATLAB Function1/4(ode4) -> Integrator b4/1
  reset1/1 -> Integrator b4/2, Integrator b3/2, Integrator b2/2, Integrator b1/2  "reset_after"
  Integrator b1/1 -> Multiport Switch/2  "integrator t1"
  Integrator b2/1 -> Multiport Switch/3  "integrator t2"
  Integrator b3/1 -> Multiport Switch/4  "integrator t3"
  Integrator b4/1 -> Multiport Switch/5
  OFF/1 -> MATLAB Function/3(OFF)
  ON/1 -> MATLAB Function/2(ON)
  xx/1 -> x/1, Scope/2, Integrator b2/3, Integrator b4/3, MATLAB Function1/1(x), MATLAB Function/4(x)
  Multiport Switch/1 -> xx/1  "x"

== system waterTankBurner/waterTank18 ==
  note: integrator t4
  ON : Inport
  OFF : Inport  Port=2
  INIT y1 : Constant  Value=20
  INIT y3 : Constant  Value=100
  Integrator b{1..4} (4 alike) : DiscreteIntegrator  ExternalReset=either  InitialConditionSource=external  InitialCondition=510  InitialConditionSetting=State (most efficient)  SampleTime=-1
  MATLAB Function : MATLAB Function  Priority=1  TreatAsAtomicUnit=on
  MATLAB Function1 : MATLAB Function  TreatAsAtomicUnit=on
  Multiport Switch : MultiPortSwitch  Inputs=4
  Scope : Scope  NumInputPorts=8
      settings: TickLabels=on  ShowLegends=on  YMin=0~0~0~0~0~0~0~0  YMax=1~1~1~1~1~1~1~1
  q : Memory  X0=1  LinearizeMemory=on
  reset1 : Memory  LinearizeMemory=on
  xx : Memory  LinearizeMemory=on
  x : Outport
  wires:
  INIT y1/1 -> Integrator b1/3
  MATLAB Function1/1(ode1) -> Integrator b1/1
  MATLAB Function/1(qNext) -> q/1  "q_before"
  q/1 -> Multiport Switch/1, MATLAB Function/1(q), Scope/1  "q_after"
  MATLAB Function/2(reset) -> reset1/1
  MATLAB Function1/2(ode2) -> Integrator b2/1
  INIT y3/1 -> Integrator b3/3
  MATLAB Function1/3(ode3) -> Integrator b3/1
  MATLAB Function1/4(ode4) -> Integrator b4/1
  reset1/1 -> Integrator b4/2, Integrator b3/2, Integrator b2/2, Integrator b1/2  "reset_after"
  Integrator b1/1 -> Multiport Switch/2  "integrator t1"
  Integrator b2/1 -> Multiport Switch/3  "integrator t2"
  Integrator b3/1 -> Multiport Switch/4  "integrator t3"
  Integrator b4/1 -> Multiport Switch/5
  OFF/1 -> MATLAB Function/3(OFF)
  ON/1 -> MATLAB Function/2(ON)
  xx/1 -> x/1, Scope/2, Integrator b2/3, Integrator b4/3, MATLAB Function1/1(x), MATLAB Function/4(x)
  Multiport Switch/1 -> xx/1  "x"

== system waterTankBurner/waterTank19 ==
  note: integrator t4
  ON : Inport
  OFF : Inport  Port=2
  INIT y1 : Constant  Value=20
  INIT y3 : Constant  Value=100
  Integrator b{1..4} (4 alike) : DiscreteIntegrator  ExternalReset=either  InitialConditionSource=external  InitialCondition=510  InitialConditionSetting=State (most efficient)  SampleTime=-1
  MATLAB Function : MATLAB Function  Priority=1  TreatAsAtomicUnit=on
  MATLAB Function1 : MATLAB Function  TreatAsAtomicUnit=on
  Multiport Switch : MultiPortSwitch  Inputs=4
  Scope : Scope  NumInputPorts=8
      settings: TickLabels=on  ShowLegends=on  YMin=0~0~0~0~0~0~0~0  YMax=1~1~1~1~1~1~1~1
  q : Memory  X0=1  LinearizeMemory=on
  reset1 : Memory  LinearizeMemory=on
  xx : Memory  LinearizeMemory=on
  x : Outport
  wires:
  INIT y1/1 -> Integrator b1/3
  MATLAB Function1/1(ode1) -> Integrator b1/1
  MATLAB Function/1(qNext) -> q/1  "q_before"
  q/1 -> Multiport Switch/1, MATLAB Function/1(q), Scope/1  "q_after"
  MATLAB Function/2(reset) -> reset1/1
  MATLAB Function1/2(ode2) -> Integrator b2/1
  INIT y3/1 -> Integrator b3/3
  MATLAB Function1/3(ode3) -> Integrator b3/1
  MATLAB Function1/4(ode4) -> Integrator b4/1
  reset1/1 -> Integrator b4/2, Integrator b3/2, Integrator b2/2, Integrator b1/2  "reset_after"
  Integrator b1/1 -> Multiport Switch/2  "integrator t1"
  Integrator b2/1 -> Multiport Switch/3  "integrator t2"
  Integrator b3/1 -> Multiport Switch/4  "integrator t3"
  Integrator b4/1 -> Multiport Switch/5
  OFF/1 -> MATLAB Function/3(OFF)
  ON/1 -> MATLAB Function/2(ON)
  xx/1 -> x/1, Scope/2, Integrator b2/3, Integrator b4/3, MATLAB Function1/1(x), MATLAB Function/4(x)
  Multiport Switch/1 -> xx/1  "x"

== system waterTankBurner/waterTank2 ==
  note: integrator t4
  ON : Inport
  OFF : Inport  Port=2
  INIT y1 : Constant  Value=20
  INIT y3 : Constant  Value=100
  Integrator b{1..4} (4 alike) : DiscreteIntegrator  ExternalReset=either  InitialConditionSource=external  InitialCondition=510  InitialConditionSetting=State (most efficient)  SampleTime=-1
  MATLAB Function : MATLAB Function  Priority=1  TreatAsAtomicUnit=on
  MATLAB Function1 : MATLAB Function  TreatAsAtomicUnit=on
  Multiport Switch : MultiPortSwitch  Inputs=4
  Scope : Scope  NumInputPorts=8
      settings: TickLabels=on  ShowLegends=on  YMin=0~0~0~0~0~0~0~0  YMax=1~1~1~1~1~1~1~1
  q : Memory  X0=1  LinearizeMemory=on
  reset1 : Memory  LinearizeMemory=on
  xx : Memory  LinearizeMemory=on
  x : Outport
  wires:
  INIT y1/1 -> Integrator b1/3
  MATLAB Function1/1(ode1) -> Integrator b1/1
  MATLAB Function/1(qNext) -> q/1  "q_before"
  q/1 -> Multiport Switch/1, MATLAB Function/1(q), Scope/1  "q_after"
  MATLAB Function/2(reset) -> reset1/1
  MATLAB Function1/2(ode2) -> Integrator b2/1
  INIT y3/1 -> Integrator b3/3
  MATLAB Function1/3(ode3) -> Integrator b3/1
  MATLAB Function1/4(ode4) -> Integrator b4/1
  reset1/1 -> Integrator b4/2, Integrator b3/2, Integrator b2/2, Integrator b1/2  "reset_after"
  Integrator b1/1 -> Multiport Switch/2  "integrator t1"
  Integrator b2/1 -> Multiport Switch/3  "integrator t2"
  Integrator b3/1 -> Multiport Switch/4  "integrator t3"
  Integrator b4/1 -> Multiport Switch/5
  OFF/1 -> MATLAB Function/3(OFF)
  ON/1 -> MATLAB Function/2(ON)
  xx/1 -> x/1, Scope/2, Integrator b2/3, Integrator b4/3, MATLAB Function1/1(x), MATLAB Function/4(x)
  Multiport Switch/1 -> xx/1  "x"

== system waterTankBurner/waterTank20 ==
  note: integrator t4
  ON : Inport
  OFF : Inport  Port=2
  INIT y1 : Constant  Value=20
  INIT y3 : Constant  Value=100
  Integrator b{1..4} (4 alike) : DiscreteIntegrator  ExternalReset=either  InitialConditionSource=external  InitialCondition=510  InitialConditionSetting=State (most efficient)  SampleTime=-1
  MATLAB Function : MATLAB Function  Priority=1  TreatAsAtomicUnit=on
  MATLAB Function1 : MATLAB Function  TreatAsAtomicUnit=on
  Multiport Switch : MultiPortSwitch  Inputs=4
  Scope : Scope  NumInputPorts=8
      settings: TickLabels=on  ShowLegends=on  YMin=0~0~0~0~0~0~0~0  YMax=1~1~1~1~1~1~1~1
  q : Memory  X0=1  LinearizeMemory=on
  reset1 : Memory  LinearizeMemory=on
  xx : Memory  LinearizeMemory=on
  x : Outport
  wires:
  INIT y1/1 -> Integrator b1/3
  MATLAB Function1/1(ode1) -> Integrator b1/1
  MATLAB Function/1(qNext) -> q/1  "q_before"
  q/1 -> Multiport Switch/1, MATLAB Function/1(q), Scope/1  "q_after"
  MATLAB Function/2(reset) -> reset1/1
  MATLAB Function1/2(ode2) -> Integrator b2/1
  INIT y3/1 -> Integrator b3/3
  MATLAB Function1/3(ode3) -> Integrator b3/1
  MATLAB Function1/4(ode4) -> Integrator b4/1
  reset1/1 -> Integrator b4/2, Integrator b3/2, Integrator b2/2, Integrator b1/2  "reset_after"
  Integrator b1/1 -> Multiport Switch/2  "integrator t1"
  Integrator b2/1 -> Multiport Switch/3  "integrator t2"
  Integrator b3/1 -> Multiport Switch/4  "integrator t3"
  Integrator b4/1 -> Multiport Switch/5
  OFF/1 -> MATLAB Function/3(OFF)
  ON/1 -> MATLAB Function/2(ON)
  xx/1 -> x/1, Scope/2, Integrator b2/3, Integrator b4/3, MATLAB Function1/1(x), MATLAB Function/4(x)
  Multiport Switch/1 -> xx/1  "x"

== system waterTankBurner/waterTank21 ==
  note: integrator t4
  ON : Inport
  OFF : Inport  Port=2
  INIT y1 : Constant  Value=20
  INIT y3 : Constant  Value=100
  Integrator b{1..4} (4 alike) : DiscreteIntegrator  ExternalReset=either  InitialConditionSource=external  InitialCondition=510  InitialConditionSetting=State (most efficient)  SampleTime=-1
  MATLAB Function : MATLAB Function  Priority=1  TreatAsAtomicUnit=on
  MATLAB Function1 : MATLAB Function  TreatAsAtomicUnit=on
  Multiport Switch : MultiPortSwitch  Inputs=4
  Scope : Scope  NumInputPorts=8
      settings: TickLabels=on  ShowLegends=on  YMin=0~0~0~0~0~0~0~0  YMax=1~1~1~1~1~1~1~1
  q : Memory  X0=1  LinearizeMemory=on
  reset1 : Memory  LinearizeMemory=on
  xx : Memory  LinearizeMemory=on
  x : Outport
  wires:
  INIT y1/1 -> Integrator b1/3
  MATLAB Function1/1(ode1) -> Integrator b1/1
  MATLAB Function/1(qNext) -> q/1  "q_before"
  q/1 -> Multiport Switch/1, MATLAB Function/1(q), Scope/1  "q_after"
  MATLAB Function/2(reset) -> reset1/1
  MATLAB Function1/2(ode2) -> Integrator b2/1
  INIT y3/1 -> Integrator b3/3
  MATLAB Function1/3(ode3) -> Integrator b3/1
  MATLAB Function1/4(ode4) -> Integrator b4/1
  reset1/1 -> Integrator b4/2, Integrator b3/2, Integrator b2/2, Integrator b1/2  "reset_after"
  Integrator b1/1 -> Multiport Switch/2  "integrator t1"
  Integrator b2/1 -> Multiport Switch/3  "integrator t2"
  Integrator b3/1 -> Multiport Switch/4  "integrator t3"
  Integrator b4/1 -> Multiport Switch/5
  OFF/1 -> MATLAB Function/3(OFF)
  ON/1 -> MATLAB Function/2(ON)
  xx/1 -> x/1, Scope/2, Integrator b2/3, Integrator b4/3, MATLAB Function1/1(x), MATLAB Function/4(x)
  Multiport Switch/1 -> xx/1  "x"

== system waterTankBurner/waterTank22 ==
  note: integrator t4
  ON : Inport
  OFF : Inport  Port=2
  INIT y1 : Constant  Value=20
  INIT y3 : Constant  Value=100
  Integrator b{1..4} (4 alike) : DiscreteIntegrator  ExternalReset=either  InitialConditionSource=external  InitialCondition=510  InitialConditionSetting=State (most efficient)  SampleTime=-1
  MATLAB Function : MATLAB Function  Priority=1  TreatAsAtomicUnit=on
  MATLAB Function1 : MATLAB Function  TreatAsAtomicUnit=on
  Multiport Switch : MultiPortSwitch  Inputs=4
  Scope : Scope  NumInputPorts=8
      settings: TickLabels=on  ShowLegends=on  YMin=0~0~0~0~0~0~0~0  YMax=1~1~1~1~1~1~1~1
  q : Memory  X0=1  LinearizeMemory=on
  reset1 : Memory  LinearizeMemory=on
  xx : Memory  LinearizeMemory=on
  x : Outport
  wires:
  INIT y1/1 -> Integrator b1/3
  MATLAB Function1/1(ode1) -> Integrator b1/1
  MATLAB Function/1(qNext) -> q/1  "q_before"
  q/1 -> Multiport Switch/1, MATLAB Function/1(q), Scope/1  "q_after"
  MATLAB Function/2(reset) -> reset1/1
  MATLAB Function1/2(ode2) -> Integrator b2/1
  INIT y3/1 -> Integrator b3/3
  MATLAB Function1/3(ode3) -> Integrator b3/1
  MATLAB Function1/4(ode4) -> Integrator b4/1
  reset1/1 -> Integrator b4/2, Integrator b3/2, Integrator b2/2, Integrator b1/2  "reset_after"
  Integrator b1/1 -> Multiport Switch/2  "integrator t1"
  Integrator b2/1 -> Multiport Switch/3  "integrator t2"
  Integrator b3/1 -> Multiport Switch/4  "integrator t3"
  Integrator b4/1 -> Multiport Switch/5
  OFF/1 -> MATLAB Function/3(OFF)
  ON/1 -> MATLAB Function/2(ON)
  xx/1 -> x/1, Scope/2, Integrator b2/3, Integrator b4/3, MATLAB Function1/1(x), MATLAB Function/4(x)
  Multiport Switch/1 -> xx/1  "x"

== system waterTankBurner/waterTank23 ==
  note: integrator t4
  ON : Inport
  OFF : Inport  Port=2
  INIT y1 : Constant  Value=20
  INIT y3 : Constant  Value=100
  Integrator b{1..4} (4 alike) : DiscreteIntegrator  ExternalReset=either  InitialConditionSource=external  InitialCondition=510  InitialConditionSetting=State (most efficient)  SampleTime=-1
  MATLAB Function : MATLAB Function  Priority=1  TreatAsAtomicUnit=on
  MATLAB Function1 : MATLAB Function  TreatAsAtomicUnit=on
  Multiport Switch : MultiPortSwitch  Inputs=4
  Scope : Scope  NumInputPorts=8
      settings: TickLabels=on  ShowLegends=on  YMin=0~0~0~0~0~0~0~0  YMax=1~1~1~1~1~1~1~1
  q : Memory  X0=1  LinearizeMemory=on
  reset1 : Memory  LinearizeMemory=on
  xx : Memory  LinearizeMemory=on
  x : Outport
  wires:
  INIT y1/1 -> Integrator b1/3
  MATLAB Function1/1(ode1) -> Integrator b1/1
  MATLAB Function/1(qNext) -> q/1  "q_before"
  q/1 -> Multiport Switch/1, MATLAB Function/1(q), Scope/1  "q_after"
  MATLAB Function/2(reset) -> reset1/1
  MATLAB Function1/2(ode2) -> Integrator b2/1
  INIT y3/1 -> Integrator b3/3
  MATLAB Function1/3(ode3) -> Integrator b3/1
  MATLAB Function1/4(ode4) -> Integrator b4/1
  reset1/1 -> Integrator b4/2, Integrator b3/2, Integrator b2/2, Integrator b1/2  "reset_after"
  Integrator b1/1 -> Multiport Switch/2  "integrator t1"
  Integrator b2/1 -> Multiport Switch/3  "integrator t2"
  Integrator b3/1 -> Multiport Switch/4  "integrator t3"
  Integrator b4/1 -> Multiport Switch/5
  OFF/1 -> MATLAB Function/3(OFF)
  ON/1 -> MATLAB Function/2(ON)
  xx/1 -> x/1, Scope/2, Integrator b2/3, Integrator b4/3, MATLAB Function1/1(x), MATLAB Function/4(x)
  Multiport Switch/1 -> xx/1  "x"

== system waterTankBurner/waterTank24 ==
  note: integrator t4
  ON : Inport
  OFF : Inport  Port=2
  INIT y1 : Constant  Value=20
  INIT y3 : Constant  Value=100
  Integrator b{1..4} (4 alike) : DiscreteIntegrator  ExternalReset=either  InitialConditionSource=external  InitialCondition=510  InitialConditionSetting=State (most efficient)  SampleTime=-1
  MATLAB Function : MATLAB Function  Priority=1  TreatAsAtomicUnit=on
  MATLAB Function1 : MATLAB Function  TreatAsAtomicUnit=on
  Multiport Switch : MultiPortSwitch  Inputs=4
  Scope : Scope  NumInputPorts=8
      settings: TickLabels=on  ShowLegends=on  YMin=0~0~0~0~0~0~0~0  YMax=1~1~1~1~1~1~1~1
  q : Memory  X0=1  LinearizeMemory=on
  reset1 : Memory  LinearizeMemory=on
  xx : Memory  LinearizeMemory=on
  x : Outport
  wires:
  INIT y1/1 -> Integrator b1/3
  MATLAB Function1/1(ode1) -> Integrator b1/1
  MATLAB Function/1(qNext) -> q/1  "q_before"
  q/1 -> Multiport Switch/1, MATLAB Function/1(q), Scope/1  "q_after"
  MATLAB Function/2(reset) -> reset1/1
  MATLAB Function1/2(ode2) -> Integrator b2/1
  INIT y3/1 -> Integrator b3/3
  MATLAB Function1/3(ode3) -> Integrator b3/1
  MATLAB Function1/4(ode4) -> Integrator b4/1
  reset1/1 -> Integrator b4/2, Integrator b3/2, Integrator b2/2, Integrator b1/2  "reset_after"
  Integrator b1/1 -> Multiport Switch/2  "integrator t1"
  Integrator b2/1 -> Multiport Switch/3  "integrator t2"
  Integrator b3/1 -> Multiport Switch/4  "integrator t3"
  Integrator b4/1 -> Multiport Switch/5
  OFF/1 -> MATLAB Function/3(OFF)
  ON/1 -> MATLAB Function/2(ON)
  xx/1 -> x/1, Scope/2, Integrator b2/3, Integrator b4/3, MATLAB Function1/1(x), MATLAB Function/4(x)
  Multiport Switch/1 -> xx/1  "x"

== system waterTankBurner/waterTank25 ==
  note: integrator t4
  ON : Inport
  OFF : Inport  Port=2
  INIT y1 : Constant  Value=20
  INIT y3 : Constant  Value=100
  Integrator b{1..4} (4 alike) : DiscreteIntegrator  ExternalReset=either  InitialConditionSource=external  InitialCondition=510  InitialConditionSetting=State (most efficient)  SampleTime=-1
  MATLAB Function : MATLAB Function  Priority=1  TreatAsAtomicUnit=on
  MATLAB Function1 : MATLAB Function  TreatAsAtomicUnit=on
  Multiport Switch : MultiPortSwitch  Inputs=4
  Scope : Scope  NumInputPorts=8
      settings: TickLabels=on  ShowLegends=on  YMin=0~0~0~0~0~0~0~0  YMax=1~1~1~1~1~1~1~1
  q : Memory  X0=1  LinearizeMemory=on
  reset1 : Memory  LinearizeMemory=on
  xx : Memory  LinearizeMemory=on
  x : Outport
  wires:
  INIT y1/1 -> Integrator b1/3
  MATLAB Function1/1(ode1) -> Integrator b1/1
  MATLAB Function/1(qNext) -> q/1  "q_before"
  q/1 -> Multiport Switch/1, MATLAB Function/1(q), Scope/1  "q_after"
  MATLAB Function/2(reset) -> reset1/1
  MATLAB Function1/2(ode2) -> Integrator b2/1
  INIT y3/1 -> Integrator b3/3
  MATLAB Function1/3(ode3) -> Integrator b3/1
  MATLAB Function1/4(ode4) -> Integrator b4/1
  reset1/1 -> Integrator b4/2, Integrator b3/2, Integrator b2/2, Integrator b1/2  "reset_after"
  Integrator b1/1 -> Multiport Switch/2  "integrator t1"
  Integrator b2/1 -> Multiport Switch/3  "integrator t2"
  Integrator b3/1 -> Multiport Switch/4  "integrator t3"
  Integrator b4/1 -> Multiport Switch/5
  OFF/1 -> MATLAB Function/3(OFF)
  ON/1 -> MATLAB Function/2(ON)
  xx/1 -> x/1, Scope/2, Integrator b2/3, Integrator b4/3, MATLAB Function1/1(x), MATLAB Function/4(x)
  Multiport Switch/1 -> xx/1  "x"

== system waterTankBurner/waterTank26 ==
  note: integrator t4
  ON : Inport
  OFF : Inport  Port=2
  INIT y1 : Constant  Value=20
  INIT y3 : Constant  Value=100
  Integrator b{1..4} (4 alike) : DiscreteIntegrator  ExternalReset=either  InitialConditionSource=external  InitialCondition=510  InitialConditionSetting=State (most efficient)  SampleTime=-1
  MATLAB Function : MATLAB Function  Priority=1  TreatAsAtomicUnit=on
  MATLAB Function1 : MATLAB Function  TreatAsAtomicUnit=on
  Multiport Switch : MultiPortSwitch  Inputs=4
  Scope : Scope  NumInputPorts=8
      settings: TickLabels=on  ShowLegends=on  YMin=0~0~0~0~0~0~0~0  YMax=1~1~1~1~1~1~1~1
  q : Memory  X0=1  LinearizeMemory=on
  reset1 : Memory  LinearizeMemory=on
  xx : Memory  LinearizeMemory=on
  x : Outport
  wires:
  INIT y1/1 -> Integrator b1/3
  MATLAB Function1/1(ode1) -> Integrator b1/1
  MATLAB Function/1(qNext) -> q/1  "q_before"
  q/1 -> Multiport Switch/1, MATLAB Function/1(q), Scope/1  "q_after"
  MATLAB Function/2(reset) -> reset1/1
  MATLAB Function1/2(ode2) -> Integrator b2/1
  INIT y3/1 -> Integrator b3/3
  MATLAB Function1/3(ode3) -> Integrator b3/1
  MATLAB Function1/4(ode4) -> Integrator b4/1
  reset1/1 -> Integrator b4/2, Integrator b3/2, Integrator b2/2, Integrator b1/2  "reset_after"
  Integrator b1/1 -> Multiport Switch/2  "integrator t1"
  Integrator b2/1 -> Multiport Switch/3  "integrator t2"
  Integrator b3/1 -> Multiport Switch/4  "integrator t3"
  Integrator b4/1 -> Multiport Switch/5
  OFF/1 -> MATLAB Function/3(OFF)
  ON/1 -> MATLAB Function/2(ON)
  xx/1 -> x/1, Scope/2, Integrator b2/3, Integrator b4/3, MATLAB Function1/1(x), MATLAB Function/4(x)
  Multiport Switch/1 -> xx/1  "x"

== system waterTankBurner/waterTank27 ==
  note: integrator t4
  ON : Inport
  OFF : Inport  Port=2
  INIT y1 : Constant  Value=20
  INIT y3 : Constant  Value=100
  Integrator b{1..4} (4 alike) : DiscreteIntegrator  ExternalReset=either  InitialConditionSource=external  InitialCondition=510  InitialConditionSetting=State (most efficient)  SampleTime=-1
  MATLAB Function : MATLAB Function  Priority=1  TreatAsAtomicUnit=on
  MATLAB Function1 : MATLAB Function  TreatAsAtomicUnit=on
  Multiport Switch : MultiPortSwitch  Inputs=4
  Scope : Scope  NumInputPorts=8
      settings: TickLabels=on  ShowLegends=on  YMin=0~0~0~0~0~0~0~0  YMax=1~1~1~1~1~1~1~1
  q : Memory  X0=1  LinearizeMemory=on
  reset1 : Memory  LinearizeMemory=on
  xx : Memory  LinearizeMemory=on
  x : Outport
  wires:
  INIT y1/1 -> Integrator b1/3
  MATLAB Function1/1(ode1) -> Integrator b1/1
  MATLAB Function/1(qNext) -> q/1  "q_before"
  q/1 -> Multiport Switch/1, MATLAB Function/1(q), Scope/1  "q_after"
  MATLAB Function/2(reset) -> reset1/1
  MATLAB Function1/2(ode2) -> Integrator b2/1
  INIT y3/1 -> Integrator b3/3
  MATLAB Function1/3(ode3) -> Integrator b3/1
  MATLAB Function1/4(ode4) -> Integrator b4/1
  reset1/1 -> Integrator b4/2, Integrator b3/2, Integrator b2/2, Integrator b1/2  "reset_after"
  Integrator b1/1 -> Multiport Switch/2  "integrator t1"
  Integrator b2/1 -> Multiport Switch/3  "integrator t2"
  Integrator b3/1 -> Multiport Switch/4  "integrator t3"
  Integrator b4/1 -> Multiport Switch/5
  OFF/1 -> MATLAB Function/3(OFF)
  ON/1 -> MATLAB Function/2(ON)
  xx/1 -> x/1, Scope/2, Integrator b2/3, Integrator b4/3, MATLAB Function1/1(x), MATLAB Function/4(x)
  Multiport Switch/1 -> xx/1  "x"

== system waterTankBurner/waterTank28 ==
  note: integrator t4
  ON : Inport
  OFF : Inport  Port=2
  INIT y1 : Constant  Value=20
  INIT y3 : Constant  Value=100
  Integrator b{1..4} (4 alike) : DiscreteIntegrator  ExternalReset=either  InitialConditionSource=external  InitialCondition=510  InitialConditionSetting=State (most efficient)  SampleTime=-1
  MATLAB Function : MATLAB Function  Priority=1  TreatAsAtomicUnit=on
  MATLAB Function1 : MATLAB Function  TreatAsAtomicUnit=on
  Multiport Switch : MultiPortSwitch  Inputs=4
  Scope : Scope  NumInputPorts=8
      settings: TickLabels=on  ShowLegends=on  YMin=0~0~0~0~0~0~0~0  YMax=1~1~1~1~1~1~1~1
  q : Memory  X0=1  LinearizeMemory=on
  reset1 : Memory  LinearizeMemory=on
  xx : Memory  LinearizeMemory=on
  x : Outport
  wires:
  INIT y1/1 -> Integrator b1/3
  MATLAB Function1/1(ode1) -> Integrator b1/1
  MATLAB Function/1(qNext) -> q/1  "q_before"
  q/1 -> Multiport Switch/1, MATLAB Function/1(q), Scope/1  "q_after"
  MATLAB Function/2(reset) -> reset1/1
  MATLAB Function1/2(ode2) -> Integrator b2/1
  INIT y3/1 -> Integrator b3/3
  MATLAB Function1/3(ode3) -> Integrator b3/1
  MATLAB Function1/4(ode4) -> Integrator b4/1
  reset1/1 -> Integrator b4/2, Integrator b3/2, Integrator b2/2, Integrator b1/2  "reset_after"
  Integrator b1/1 -> Multiport Switch/2  "integrator t1"
  Integrator b2/1 -> Multiport Switch/3  "integrator t2"
  Integrator b3/1 -> Multiport Switch/4  "integrator t3"
  Integrator b4/1 -> Multiport Switch/5
  OFF/1 -> MATLAB Function/3(OFF)
  ON/1 -> MATLAB Function/2(ON)
  xx/1 -> x/1, Scope/2, Integrator b2/3, Integrator b4/3, MATLAB Function1/1(x), MATLAB Function/4(x)
  Multiport Switch/1 -> xx/1  "x"

== system waterTankBurner/waterTank29 ==
  note: integrator t4
  ON : Inport
  OFF : Inport  Port=2
  INIT y1 : Constant  Value=20
  INIT y3 : Constant  Value=100
  Integrator b{1..4} (4 alike) : DiscreteIntegrator  ExternalReset=either  InitialConditionSource=external  InitialCondition=510  InitialConditionSetting=State (most efficient)  SampleTime=-1
  MATLAB Function : MATLAB Function  Priority=1  TreatAsAtomicUnit=on
  MATLAB Function1 : MATLAB Function  TreatAsAtomicUnit=on
  Multiport Switch : MultiPortSwitch  Inputs=4
  Scope : Scope  NumInputPorts=8
      settings: TickLabels=on  ShowLegends=on  YMin=0~0~0~0~0~0~0~0  YMax=1~1~1~1~1~1~1~1
  q : Memory  X0=1  LinearizeMemory=on
  reset1 : Memory  LinearizeMemory=on
  xx : Memory  LinearizeMemory=on
  x : Outport
  wires:
  INIT y1/1 -> Integrator b1/3
  MATLAB Function1/1(ode1) -> Integrator b1/1
  MATLAB Function/1(qNext) -> q/1  "q_before"
  q/1 -> Multiport Switch/1, MATLAB Function/1(q), Scope/1  "q_after"
  MATLAB Function/2(reset) -> reset1/1
  MATLAB Function1/2(ode2) -> Integrator b2/1
  INIT y3/1 -> Integrator b3/3
  MATLAB Function1/3(ode3) -> Integrator b3/1
  MATLAB Function1/4(ode4) -> Integrator b4/1
  reset1/1 -> Integrator b4/2, Integrator b3/2, Integrator b2/2, Integrator b1/2  "reset_after"
  Integrator b1/1 -> Multiport Switch/2  "integrator t1"
  Integrator b2/1 -> Multiport Switch/3  "integrator t2"
  Integrator b3/1 -> Multiport Switch/4  "integrator t3"
  Integrator b4/1 -> Multiport Switch/5
  OFF/1 -> MATLAB Function/3(OFF)
  ON/1 -> MATLAB Function/2(ON)
  xx/1 -> x/1, Scope/2, Integrator b2/3, Integrator b4/3, MATLAB Function1/1(x), MATLAB Function/4(x)
  Multiport Switch/1 -> xx/1  "x"

== system waterTankBurner/waterTank3 ==
  note: integrator t4
  ON : Inport
  OFF : Inport  Port=2
  INIT y1 : Constant  Value=20
  INIT y3 : Constant  Value=100
  Integrator b{1..4} (4 alike) : DiscreteIntegrator  ExternalReset=either  InitialConditionSource=external  InitialCondition=510  InitialConditionSetting=State (most efficient)  SampleTime=-1
  MATLAB Function : MATLAB Function  Priority=1  TreatAsAtomicUnit=on
  MATLAB Function1 : MATLAB Function  TreatAsAtomicUnit=on
  Multiport Switch : MultiPortSwitch  Inputs=4
  Scope : Scope  NumInputPorts=8
      settings: TickLabels=on  ShowLegends=on  YMin=0~0~0~0~0~0~0~0  YMax=1~1~1~1~1~1~1~1
  q : Memory  X0=1  LinearizeMemory=on
  reset1 : Memory  LinearizeMemory=on
  xx : Memory  LinearizeMemory=on
  x : Outport
  wires:
  INIT y1/1 -> Integrator b1/3
  MATLAB Function1/1(ode1) -> Integrator b1/1
  MATLAB Function/1(qNext) -> q/1  "q_before"
  q/1 -> Multiport Switch/1, MATLAB Function/1(q), Scope/1  "q_after"
  MATLAB Function/2(reset) -> reset1/1
  MATLAB Function1/2(ode2) -> Integrator b2/1
  INIT y3/1 -> Integrator b3/3
  MATLAB Function1/3(ode3) -> Integrator b3/1
  MATLAB Function1/4(ode4) -> Integrator b4/1
  reset1/1 -> Integrator b4/2, Integrator b3/2, Integrator b2/2, Integrator b1/2  "reset_after"
  Integrator b1/1 -> Multiport Switch/2  "integrator t1"
  Integrator b2/1 -> Multiport Switch/3  "integrator t2"
  Integrator b3/1 -> Multiport Switch/4  "integrator t3"
  Integrator b4/1 -> Multiport Switch/5
  OFF/1 -> MATLAB Function/3(OFF)
  ON/1 -> MATLAB Function/2(ON)
  xx/1 -> x/1, Scope/2, Integrator b2/3, Integrator b4/3, MATLAB Function1/1(x), MATLAB Function/4(x)
  Multiport Switch/1 -> xx/1  "x"

== system waterTankBurner/waterTank30 ==
  note: integrator t4
  ON : Inport
  OFF : Inport  Port=2
  INIT y1 : Constant  Value=20
  INIT y3 : Constant  Value=100
  Integrator b{1..4} (4 alike) : DiscreteIntegrator  ExternalReset=either  InitialConditionSource=external  InitialCondition=510  InitialConditionSetting=State (most efficient)  SampleTime=-1
  MATLAB Function : MATLAB Function  Priority=1  TreatAsAtomicUnit=on
  MATLAB Function1 : MATLAB Function  TreatAsAtomicUnit=on
  Multiport Switch : MultiPortSwitch  Inputs=4
  Scope : Scope  NumInputPorts=8
      settings: TickLabels=on  ShowLegends=on  YMin=0~0~0~0~0~0~0~0  YMax=1~1~1~1~1~1~1~1
  q : Memory  X0=1  LinearizeMemory=on
  reset1 : Memory  LinearizeMemory=on
  xx : Memory  LinearizeMemory=on
  x : Outport
  wires:
  INIT y1/1 -> Integrator b1/3
  MATLAB Function1/1(ode1) -> Integrator b1/1
  MATLAB Function/1(qNext) -> q/1  "q_before"
  q/1 -> Multiport Switch/1, MATLAB Function/1(q), Scope/1  "q_after"
  MATLAB Function/2(reset) -> reset1/1
  MATLAB Function1/2(ode2) -> Integrator b2/1
  INIT y3/1 -> Integrator b3/3
  MATLAB Function1/3(ode3) -> Integrator b3/1
  MATLAB Function1/4(ode4) -> Integrator b4/1
  reset1/1 -> Integrator b4/2, Integrator b3/2, Integrator b2/2, Integrator b1/2  "reset_after"
  Integrator b1/1 -> Multiport Switch/2  "integrator t1"
  Integrator b2/1 -> Multiport Switch/3  "integrator t2"
  Integrator b3/1 -> Multiport Switch/4  "integrator t3"
  Integrator b4/1 -> Multiport Switch/5
  OFF/1 -> MATLAB Function/3(OFF)
  ON/1 -> MATLAB Function/2(ON)
  xx/1 -> x/1, Scope/2, Integrator b2/3, Integrator b4/3, MATLAB Function1/1(x), MATLAB Function/4(x)
  Multiport Switch/1 -> xx/1  "x"
